simulink model "P4p2"  (Simulink 8.3)
settings: Solver=ode1  StartTime=0.0  StopTime=inf  FixedStep=0.002  RelTol=1e-3
PostLoadFcn:
  | qc_set_target_type(getConfigSet(bdroot, 'QUARC Default Target Configuration'));
values from neighbouring files (symbols this model uses):
  A_est = [0 1 0 0 0 0 ... (first row only)    [P4p2_init.m]    (also in P4p2_integral_init.m; P4p3_init.m)
  B_est = [0 0 ... (first row only)    [P4p2_init.m]    (also in P4p2_integral_init.m; P4p3_init.m)
  C_est = [1 0 0 0 0 0 ... (first row only)    [P4p2_init.m]    (also in P4p2_integral_init.m; P4p3_init.m)
  Joystick_gain_x = 0.8    [P4p2_init.m]    (also in P4p2_integral_init.m; P4p3_init.m)
  Joystick_gain_y = -1    [P4p2_init.m]    (also in P4p2_integral_init.m; P4p3_init.m)
  K = lqr(A, B, Q, R)    [P4p2_init.m]
  L = place(A_est.', C_est.', pol_est).'    [P4p2_init.m]    (also in P4p2_integral_init.m; P4p3_init.m = 41.406 * place(A_est.', C_est2.', pol_est).')
  P_p = inv(C * inv(B*K - A) * B)    [P4p2_init.m]
undefined symbols (not defined in the file or in its folder): Elevation_offset, HIL, Pitch_offset, qc_get_step_size, Travel_offset, V_s_meas
libraries: simulink_extras x6, quarc_library x4
settings Model: Creator=Rchan  LastModifiedBy=bendia  SimulationMode=external  ExtModeTrigDuration=5000
settings SolverCC: PositivePriorityOrder=on
settings OptimizationCC: ExpressionDepthLimit=2147483647  InitFltsAndDblsToZero=on
settings DebuggingCC: SaveWithParameterizedLinksMsg=none  MultiTaskDSMMsg=warning  MultiTaskCondExecSysMsg=none  FcnCallInpInsideContextMsg=UseLocalSettings
settings RTWCC: SystemTargetFile=quarc_win64.tlc  TemplateMakefile=quarc_default_tmf  Description=QUARC Win64 Target  ProcessScript=quarc_win64_make_rtw_hook
settings STFCustomTargetCC: TargetPreCompLibLocation=C:\PROGRA~3\QUARC\lib\2014a\win64\release  ConcurrentExecutionCompliant=on  GeneratePreprocessorConditionals=Disable all  CPPClassGenCompliant=on  SystemTargetFile=quarc_win64.tlc
settings GRTTargetCC: TargetPreCompLibLocation=C:\PROGRA~3\QUARC\lib\2014a\win64\release  ParMdlRefBuildCompliant=off  CompOptLevelCompliant=off  MatFileLogging=off  ExtMode=on  ExtModeMexFile=quarc_comm

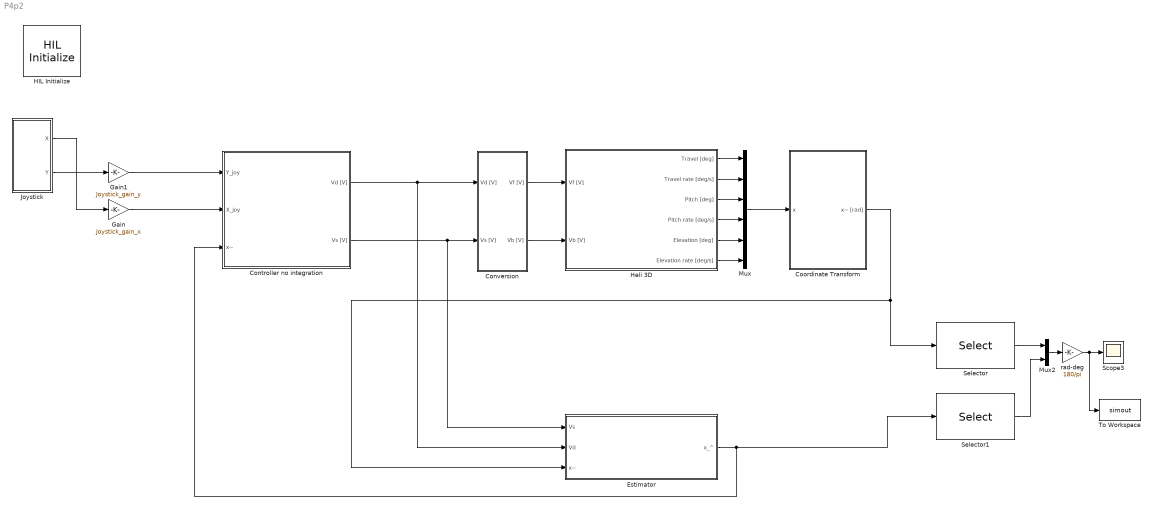
== system P4p2 ==
  Controller no integration : Subsystem
  Conversion : Subsystem
  Coordinate Transform : Subsystem
  Estimator : Subsystem
  Gain : Gain  Gain=Joystick_gain_x
  Gain1 : Gain  Gain=Joystick_gain_y
  HIL Initialize : quarc_library/Data Acquisition/Generic/Configuration/HIL Initialize  Priority=-99  object_name=HIL-1  board_type=q8_usb  board_number=0  board_options=update_rate=normal;decimation=1  exclusive=off  active=off  hardware_clocks=[0:2]  clock_modes=[]  initial_clock_frequencies=[]  set_clock_params_at_start=off  set_clock_params_at_switch_in=off  set_clock_frequencies_at_start=off  set_clock_frequencies_at_switch_in=off  analog_input_channels=[0:7]  analog_input_maximums=10  analog_input_minimums=-10  set_analog_input_params_at_start=on  set_analog_input_params_at_switch_in=off  analog_output_channels=[0:7]  analog_output_maximums=10  analog_output_minimums=-10  initial_analog_outputs=[0]  final_analog_outputs=[0]  watchdog_analog_outputs=0  set_analog_output_params_at_start=on  set_analog_output_params_at_switch_in=off  set_analog_outputs_at_start=on  set_analog_outputs_at_switch_in=off  set_analog_outputs_at_terminate=on  set_analog_outputs_at_switch_out=off  set_analog_outputs_on_watchdog=off  digital_input_channels=[]  digital_output_channels=[]  digital_output_configuration=[]  initial_digital_outputs=[1]  final_digital_outputs=[1]  watchdog_digital_outputs=[1]  set_digital_output_params_at_start=off  set_digital_output_params_at_switch_in=off  set_digital_outputs_at_start=on  set_digital_outputs_at_switch_in=off  set_digital_outputs_at_terminate=on  set_digital_outputs_at_switch_out=off  set_digital_outputs_on_watchdog=off  encoder_channels=[0:7]  quadrature=[4]  encoder_filter_frequency=[]  initial_encoder_counts=[0]  set_encoder_params_at_start=on  set_encoder_params_at_switch_in=off  set_encoder_counts_at_start=on  set_encoder_counts_at_switch_in=off  pwm_channels=[0:7]  pwm_modes=0  pwm_frequency=99.532799999999995e6/4095  pwm_configuration=[0]  pwm_alignment=[0]  pwm_polarity=[1]  pwm_leading_deadband=[0]  pwm_trailing_deadband=[0]  initial_pwm_outputs=[0]  final_pwm_outputs=[0]  watchdog_pwm_outputs=[0]  set_pwm_params_at_start=on  set_pwm_params_at_switch_in=off  set_pwm_outputs_at_start=on  set_pwm_outputs_at_switch_in=off  set_pwm_outputs_at_terminate=on  set_pwm_outputs_at_switch_out=off  set_pwm_outputs_on_watchdog=off  other_output_channels=[]  initial_other_outputs=[]  final_other_outputs=[]  watchdog_other_outputs=[]  set_other_outputs_at_start=off  set_other_outputs_at_switch_in=off  set_other_outputs_at_terminate=off  set_other_outputs_at_switch_out=off  set_other_outputs_on_watchdog=off
  Heli 3D : Subsystem
  Joystick : Subsystem
  Mux : Mux  Inputs=6
  Mux2 : Mux  Inputs=2
  Scope3 : Scope
      settings: TimeRange=10  YMin=-200  YMax=550  SaveName=ScopeData3
  Selector : Selector  InputPortWidth=6  Indices=3
  Selector1 : Selector  InputPortWidth=6  Indices=3
  To Workspace : ToWorkspace  VariableName=simout  SaveFormat=Structure With Time  SampleTime=-1
  rad-deg : Gain  Gain=180/pi
  wires:
  Conversion/2(Vb [V]) -> Heli 3D/2(Vb [V])
  Conversion/1(Vf [V]) -> Heli 3D/1(Vf [V])
  Heli 3D/1(Travel [deg]) -> Mux/1
  Heli 3D/2(Travel rate [deg/s]) -> Mux/2
  Heli 3D/3(Pitch [deg]) -> Mux/3
  Heli 3D/4(Pitch rate [deg/s]) -> Mux/4
  Heli 3D/5(Elevation [deg]) -> Mux/5
  Heli 3D/6(Elevation rate [deg/s]) -> Mux/6
  Joystick/1(X) -> Gain/1
  Joystick/2(Y) -> Gain1/1
  Mux/1 -> Coordinate Transform/1(x)
  Coordinate Transform/1(x~ [rad]) -> Selector/1, Estimator/3(x~)
  Gain/1 -> Controller no integration/2(X_joy)
  Gain1/1 -> Controller no integration/1(Y_joy)
  Controller no integration/1(Vd [V]) -> Estimator/2(Vd), Conversion/1(Vd [V])
  Controller no integration/2(Vs [V]) -> Estimator/1(Vs), Conversion/2(Vs [V])
  Mux2/1 -> rad-deg/1
  Selector/1 -> Mux2/1
  Selector1/1 -> Mux2/2
  rad-deg/1 -> To Workspace/1, Scope3/1
  Estimator/1(x_^) -> Controller no integration/3(x~), Selector1/1

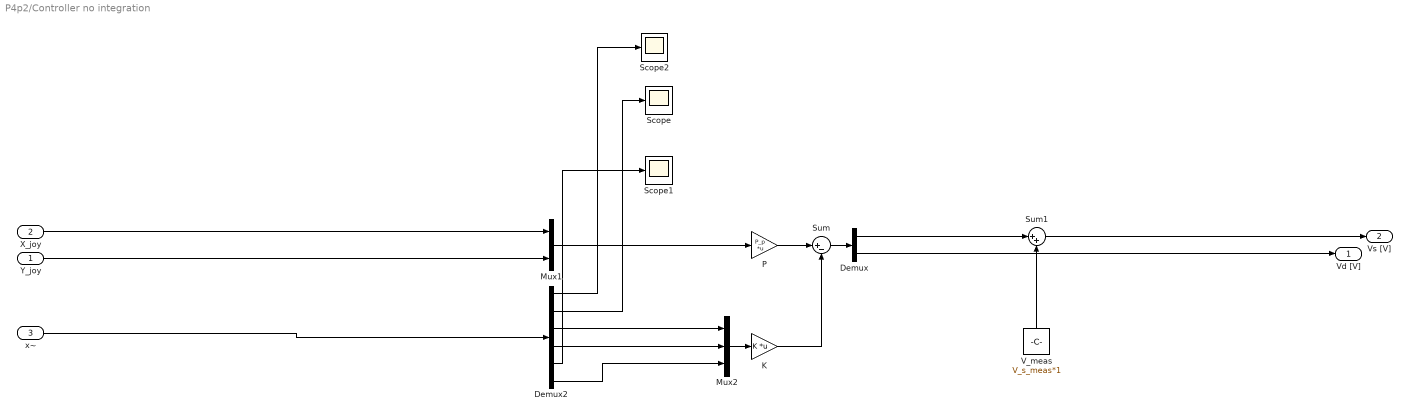
== system P4p2/Controller no integration ==
  Y_joy : Inport
  X_joy : Inport  Port=2
  x~ : Inport  Port=3
  Demux : Demux  Outputs=2
  Demux2 : Demux  Outputs=6
  K : Gain  Gain=K  Multiplication=Matrix(K*u)
  Mux1 : Mux  Inputs=2
  Mux2 : Mux  Inputs=3
  P : Gain  Gain=P_p  Multiplication=Matrix(K*u)
  Scope : Scope
      settings: SaveName=ScopeData4
  Scope1 : Scope
      settings: SaveName=ScopeData6
  Scope2 : Scope
      settings: SaveName=ScopeData14
  Sum : Sum  Inputs=|+-
  Sum1 : Sum  Inputs=|++
  V_meas : Constant  Value=V_s_meas*1
  Vd [V] : Outport
  Vs [V] : Outport  Port=2
  wires:
  x~/1 -> Demux2/1
  X_joy/1 -> Mux1/1
  P/1 -> Sum/1
  Mux1/1 -> P/1
  K/1 -> Sum/2
  Mux2/1 -> K/1
  Sum/1 -> Demux/1
  Demux/1 -> Sum1/1
  Demux/2 -> Vd [V]/1
  Sum1/1 -> Vs [V]/1
  V_meas/1 -> Sum1/2
  Demux2/3 -> Mux2/1
  Demux2/6 -> Mux2/3
  Demux2/4 -> Mux2/2
  Y_joy/1 -> Mux1/2
  Demux2/1 -> Scope2/1
  Demux2/2 -> Scope/1
  Demux2/5 -> Scope1/1

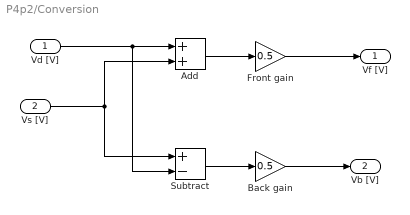
== system P4p2/Conversion ==
  Vd [V] : Inport
  Vs [V] : Inport  Port=2
  Add : Sum
  Back gain : Gain  Gain=0.5
  Front gain : Gain  Gain=0.5
  Subtract : Sum  Inputs=+-
  Vf [V] : Outport
  Vb [V] : Outport  Port=2
  wires:
  Vd [V]/1 -> Subtract/2, Add/1
  Vs [V]/1 -> Subtract/1, Add/2
  Subtract/1 -> Back gain/1
  Back gain/1 -> Vb [V]/1
  Add/1 -> Front gain/1
  Front gain/1 -> Vf [V]/1

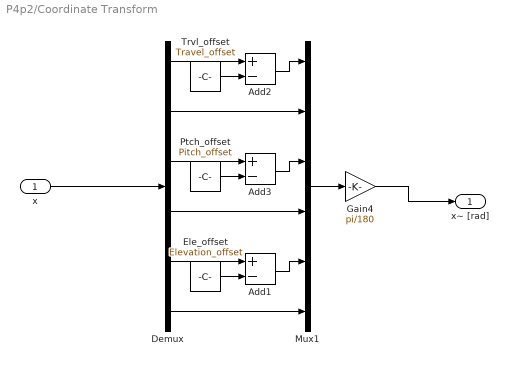
== system P4p2/Coordinate Transform ==
  x : Inport
  Add1 : Sum  Inputs=+-
  Add2 : Sum  Inputs=+-
  Add3 : Sum  Inputs=+-
  Demux : Demux  Outputs=6
  Ele_offset : Constant  Value=Elevation_offset
  Gain4 : Gain  Gain=pi/180
  Mux1 : Mux  Inputs=6
  Ptch_offset : Constant  Value=Pitch_offset
  Trvl_offset : Constant  Value=Travel_offset
  x~ [rad] : Outport
  wires:
  Demux/3 -> Add3/1
  Demux/5 -> Add1/1
  Demux/6 -> Mux1/6
  Mux1/1 -> Gain4/1
  Demux/1 -> Add2/1
  Ptch_offset/1 -> Add3/2
  Trvl_offset/1 -> Add2/2
  Gain4/1 -> x~ [rad]/1
  Ele_offset/1 -> Add1/2
  Add3/1 -> Mux1/3
  x/1 -> Demux/1
  Add1/1 -> Mux1/5
  Add2/1 -> Mux1/1
  Demux/4 -> Mux1/4
  Demux/2 -> Mux1/2

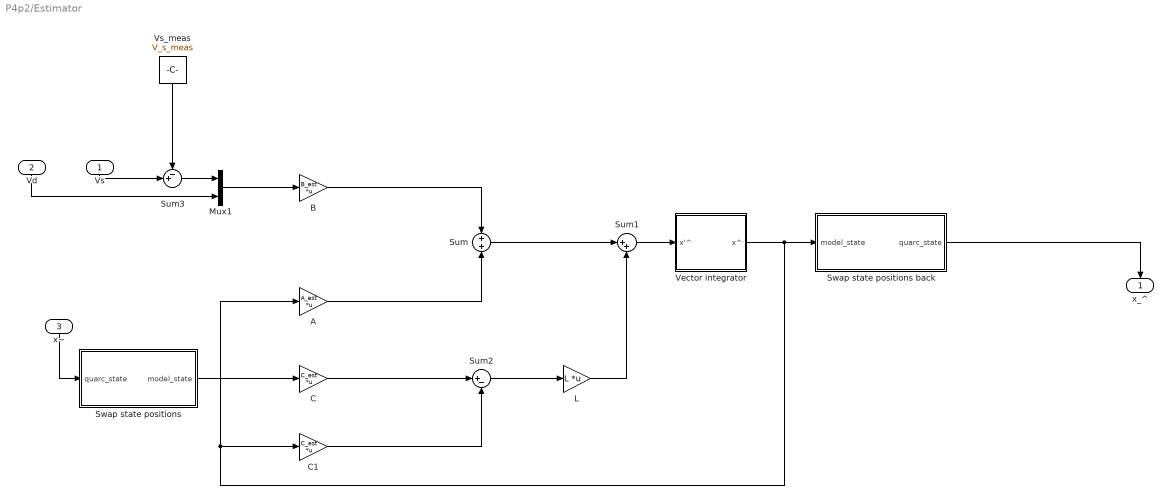
== system P4p2/Estimator ==
  Vs : Inport
  Vd : Inport  Port=2
  x~ : Inport  Port=3
  A : Gain  Gain=A_est  Multiplication=Matrix(K*u)
  B : Gain  Gain=B_est  Multiplication=Matrix(K*u)
  C : Gain  Gain=C_est  Multiplication=Matrix(K*u)
  C1 : Gain  Gain=C_est  Multiplication=Matrix(K*u)
  L : Gain  Gain=L  Multiplication=Matrix(K*u)
  Mux1 : Mux  Inputs=2
  Sum : Sum  Inputs=+|+
  Sum1 : Sum  Inputs=|++
  Sum2 : Sum  Inputs=|+-
  Sum3 : Sum  Inputs=-+|
  Swap state positions : Subsystem
  Swap state positions back : Subsystem
  Vector integrator : Subsystem
  Vs_meas : Constant  Value=V_s_meas
  x_^ : Outport
  wires:
  C/1 -> Sum2/1
  Mux1/1 -> B/1
  C1/1 -> Sum2/2
  L/1 -> Sum1/2
  Sum/1 -> Sum1/1
  Sum2/1 -> L/1
  B/1 -> Sum/1
  Vd/1 -> Mux1/2
  Sum1/1 -> Vector integrator/1(x'^)
  A/1 -> Sum/2
  Vector integrator/1(x^) -> Swap state positions back/1(model_state), C1/1, A/1
  Swap state positions/1(model_state) -> C/1
  x~/1 -> Swap state positions/1(quarc_state)
  Swap state positions back/1(quarc_state) -> x_^/1
  Vs/1 -> Sum3/2
  Sum3/1 -> Mux1/1
  Vs_meas/1 -> Sum3/1

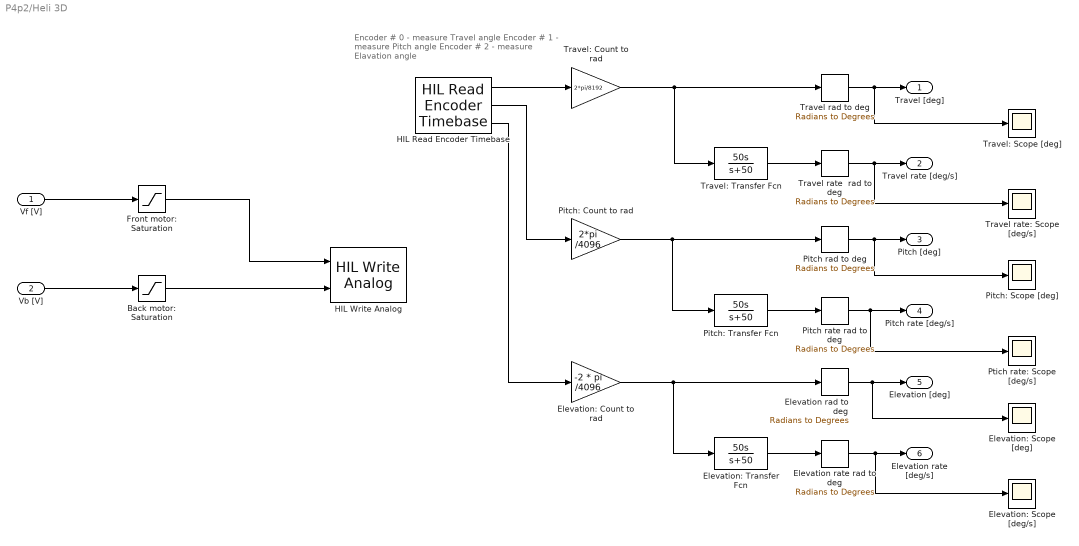
== system P4p2/Heli 3D ==
  note: Encoder # 0 - measure Travel angle
      | Encoder # 1 - measure Pitch angle
      | Encoder # 2 - measure Elavation angle
  Vf [V] : Inport
  Vb [V] : Inport  Port=2
  Back motor: Saturation : Saturate  UpperLimit=5  LowerLimit=-5
  Elevation rad to deg : simulink_extras/Transformations/Radians to Degrees
  Elevation rate rad to deg : simulink_extras/Transformations/Radians to Degrees
  Elevation: Count to rad : Gain  Gain=-2 * pi /4096
  Elevation: Scope [deg/s] : Scope
      settings: YMin=-15  YMax=15  SaveName=ScopeData13
  Elevation: Scope [deg] : Scope
      settings: YMin=-0  YMax=30  SaveName=ScopeData12
  Elevation: Transfer Fcn : TransferFcn  Numerator=[50 0]  Denominator=[1 50]
  Front motor: Saturation : Saturate  UpperLimit=5  LowerLimit=-5
  HIL Read Encoder Timebase : quarc_library/Data Acquisition/Generic/Timebases/HIL Read Encoder Timebase  object_name=HIL-1  clock=0  channels=[0:2]  samples_in_buffer=max(ceil(1/qc_get_step_size), 1)  active=on  vector_output=off  data_type_mode=Inherit via back propagation  data_type=double
  HIL Write Analog : quarc_library/Data Acquisition/Generic/Immediate I//O/HIL Write Analog  object_name=HIL-1  channels=[0:1]  sample_time=-1  active=off  vector_input=off
  Pitch rad to deg : simulink_extras/Transformations/Radians to Degrees
  Pitch rate rad to deg : simulink_extras/Transformations/Radians to Degrees
  Pitch: Count to rad : Gain  Gain=2*pi /4096
  Pitch: Scope [deg] : Scope
      settings: YMin=-15  YMax=15  SaveName=ScopeData10
  Pitch: Transfer Fcn : TransferFcn  Numerator=[50 0]  Denominator=[1 50]
  Ptich rate: Scope [deg/s] : Scope
      settings: YMin=-15  YMax=15  SaveName=ScopeData11
  Travel rad to deg : simulink_extras/Transformations/Radians to Degrees
  Travel rate  rad to deg : simulink_extras/Transformations/Radians to Degrees
  Travel rate: Scope [deg/s] : Scope
      settings: YMin=-15  YMax=15  SaveName=ScopeData9
  Travel: Count to rad : Gain  Gain=2*pi/8192
  Travel: Scope [deg] : Scope
      settings: YMin=-15  YMax=15  SaveName=ScopeData8
  Travel: Transfer Fcn : TransferFcn  Numerator=[50 0]  Denominator=[1 50]
  Travel [deg] : Outport
  Travel rate [deg/s] : Outport  Port=2
  Pitch [deg] : Outport  Port=3
  Pitch rate [deg/s] : Outport  Port=4
  Elevation [deg] : Outport  Port=5
  Elevation rate [deg/s] : Outport  Port=6
  wires:
  HIL Read Encoder Timebase/1 -> Travel: Count to rad/1
  HIL Read Encoder Timebase/2 -> Pitch: Count to rad/1
  HIL Read Encoder Timebase/3 -> Elevation: Count to rad/1
  Travel: Count to rad/1 -> Travel: Transfer Fcn/1, Travel rad to deg/1
  Travel: Transfer Fcn/1 -> Travel rate  rad to deg/1
  Pitch: Count to rad/1 -> Pitch: Transfer Fcn/1, Pitch rad to deg/1
  Pitch: Transfer Fcn/1 -> Pitch rate rad to deg/1
  Elevation: Count to rad/1 -> Elevation: Transfer Fcn/1, Elevation rad to deg/1
  Elevation: Transfer Fcn/1 -> Elevation rate rad to deg/1
  Travel rad to deg/1 -> Travel: Scope [deg]/1, Travel [deg]/1
  Travel rate  rad to deg/1 -> Travel rate: Scope [deg/s]/1, Travel rate [deg/s]/1
  Pitch rad to deg/1 -> Pitch: Scope [deg]/1, Pitch [deg]/1
  Pitch rate rad to deg/1 -> Ptich rate: Scope [deg/s]/1, Pitch rate [deg/s]/1
  Elevation rad to deg/1 -> Elevation: Scope [deg]/1, Elevation [deg]/1
  Elevation rate rad to deg/1 -> Elevation: Scope [deg/s]/1, Elevation rate [deg/s]/1
  Vf [V]/1 -> Front motor: Saturation/1
  Vb [V]/1 -> Back motor: Saturation/1
  Front motor: Saturation/1 -> HIL Write Analog/1
  Back motor: Saturation/1 -> HIL Write Analog/2

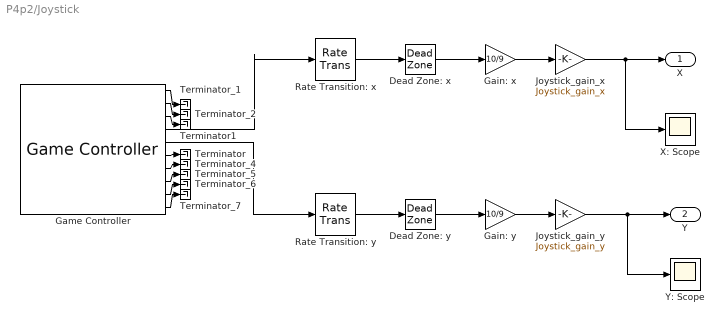
== system P4p2/Joystick ==
  Dead Zone: x : DeadZone  LowerValue=-0.1  UpperValue=0.1  SaturateOnIntegerOverflow=on
  Dead Zone: y : DeadZone  LowerValue=-0.1  UpperValue=0.1  SaturateOnIntegerOverflow=on
  Gain: x : Gain  Gain=10/9
  Gain: y : Gain  Gain=10/9
  Game Controller : quarc_library/Devices/Peripherals/Target/Game Controller  controller=1  buffer_size=12  deadzone=[]  saturation=[]  sample_time=max(qc_get_step_size, 0.01)  auto_center=off  enabled=on
  Joystick_gain_x : Gain  Gain=Joystick_gain_x
  Joystick_gain_y : Gain  Gain=Joystick_gain_y
  Rate Transition: x : RateTransition
  Rate Transition: y : RateTransition
  Terminator : Terminator
  Terminator1 : Terminator
  Terminator_{1..2,4..7} (6 alike) : Terminator
  X: Scope : Scope
      settings: YMin=-1  YMax=1  SaveName=ScopeData7
  Y: Scope : Scope
      settings: YMin=-10  YMax=10  SaveName=ScopeData5
  X : Outport
  Y : Outport  Port=2
  wires:
  Rate Transition: y/1 -> Dead Zone: y/1
  Rate Transition: x/1 -> Dead Zone: x/1
  Game Controller/5 -> Rate Transition: y/1
  Game Controller/4 -> Rate Transition: x/1
  Game Controller/1 -> Terminator_1/1
  Game Controller/2 -> Terminator_2/1
  Game Controller/7 -> Terminator_4/1
  Game Controller/8 -> Terminator_5/1
  Game Controller/9 -> Terminator_6/1
  Game Controller/10 -> Terminator_7/1
  Game Controller/3 -> Terminator1/1
  Game Controller/6 -> Terminator/1
  Dead Zone: x/1 -> Gain: x/1
  Dead Zone: y/1 -> Gain: y/1
  Gain: x/1 -> Joystick_gain_x/1
  Gain: y/1 -> Joystick_gain_y/1
  Joystick_gain_x/1 -> X/1, X: Scope/1
  Joystick_gain_y/1 -> Y: Scope/1, Y/1

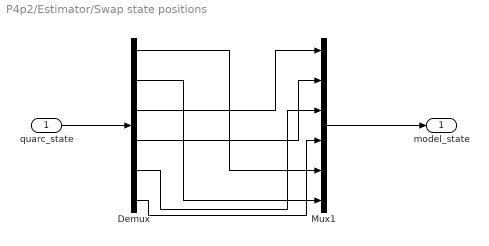
== system P4p2/Estimator/Swap state positions ==
  quarc_state : Inport
  Demux : Demux  Outputs=6
  Mux1 : Mux  Inputs=6
  model_state : Outport
  wires:
  Demux/1 -> Mux1/5
  Mux1/1 -> model_state/1
  Demux/3 -> Mux1/1
  Demux/5 -> Mux1/3
  quarc_state/1 -> Demux/1
  Demux/6 -> Mux1/4
  Demux/4 -> Mux1/2
  Demux/2 -> Mux1/6

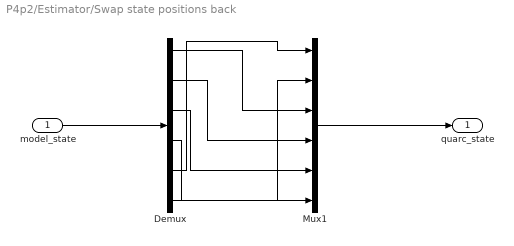
== system P4p2/Estimator/Swap state positions back ==
  model_state : Inport
  Demux : Demux  Outputs=6
  Mux1 : Mux  Inputs=6
  quarc_state : Outport
  wires:
  Demux/2 -> Mux1/4
  Mux1/1 -> quarc_state/1
  Demux/4 -> Mux1/6
  Demux/5 -> Mux1/1
  model_state/1 -> Demux/1
  Demux/1 -> Mux1/3
  Demux/3 -> Mux1/5
  Demux/6 -> Mux1/2

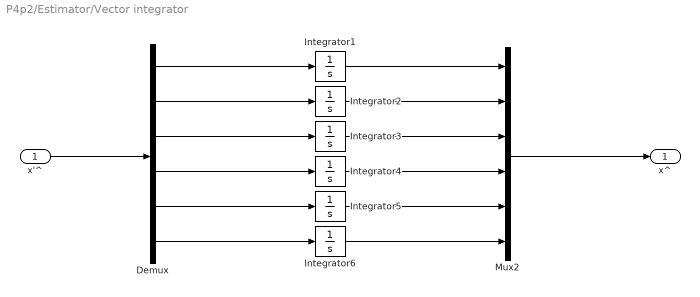
== system P4p2/Estimator/Vector integrator ==
  x'^ : Inport
  Demux : Demux  Outputs=6
  Integrator{1..6} (6 alike) : Integrator
  Mux2 : Mux  Inputs=6
  x^ : Outport
  wires:
  Integrator1/1 -> Mux2/1
  Demux/1 -> Integrator1/1
  Demux/5 -> Integrator5/1
  x'^/1 -> Demux/1
  Integrator2/1 -> Mux2/2
  Demux/2 -> Integrator2/1
  Demux/4 -> Integrator4/1
  Mux2/1 -> x^/1
  Demux/6 -> Integrator6/1
  Integrator3/1 -> Mux2/3
  Integrator6/1 -> Mux2/6
  Integrator5/1 -> Mux2/5
  Demux/3 -> Integrator3/1
  Integrator4/1 -> Mux2/4
